simulink library "dspvect2"  (Simulink 3.00)
libraries: dspvect2 x2
settings Model: Creator=don  LastModifiedBy=tjones

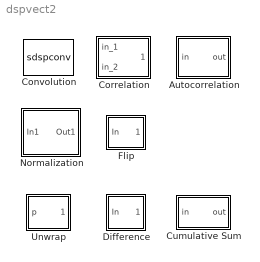
== system dspvect2 ==
  Autocorrelation : Subsystem  mask(Autocorrelation){maxlag=-1, bias=None}
      mask prompts: maxlag "Maximum positive lag (-1 for all positive lags)"; bias "Scaling:"
      mask help: Computes the autocorrelation function for non-negative lags in the range [0, length(u)-1].
      mask Help: web(dspbhelp);
      mask StyleString: edit,popup(None|Biased|Unbiased|Unity at zero-lag)
      mask Display: disp('ACF')
  Convolution : S-Function  FunctionName=sdspconv  PortCounts=[]  SFunctionModules=''
      mask Type: Convolution
      mask Description: Convolve two vectors.
      mask Help: web(dspbhelp);
      mask Display: disp('Conv')
  Correlation : Subsystem
      mask Type: Correlation
      mask Description: Correlation between two vectors.
      mask Help: web(dspbhelp);
      mask Display: disp('Corr')
  Cumulative Sum : Subsystem
      mask Type: Cumulative Sum
      mask Description: Cumulative sum of input elements.
      mask Help: web(dspbhelp);
      mask Display: disp('cumsum')
  Difference : Subsystem
      mask Type: Difference
      mask Description: Difference between adjacent vector input elements.
      mask Help: web(dspbhelp);
      mask Display: disp('diff')
  Flip : Subsystem
      mask Type: Flip
      mask Description: Reverse order of vector elements.
      mask Help: web(dspbhelp);
      mask Display: plot(0,0,100,100,[47 40 40 47],[20 20 90 90],[53 60 60 53],[90 90 20 20],[75 76 81 80 73],[34 24 40 60 90],[83 76],[29 24],[19 30 19 19 26],[86 84 72 50 20],[29 30],[71 84])
  Normalization : Subsystem  mask(Normalization){NormType=Squared 2-norm, Bias=1e-10}
      mask prompts: NormType "Norm:"; Bias "Normalization bias:"
      mask help: Normalize each input element by the vector 2-norm, sqrt(u'u)+b, or by the squared 2-norm, u'u+b, where b is a bias used to protect against divide-by-zero.
      mask init:
      | x = [0 NaN 100 NaN 20 80 NaN 30 30 NaN 36 36 NaN 58 58 NaN 64 64];
      | y = [0 NaN 100 NaN 60 60 NaN 9 43 NaN 9 43 NaN 9 43 NaN 9 43];
      | if NormType==1, sqr_txt = ' '; else sqr_txt = '2'; end
      mask Help: web(dspbhelp);
      mask StyleString: popup(2-norm|Squared 2-norm),edit
      mask Display:
      | plot(x,y)
      | text(44,80,'u'); text(44,25,'u'); text(72,39,sqr_txt)
  Unwrap : Subsystem  mask(Unwrap){tol=pi}
      mask prompts: tol "Tolerance (radians):"
      mask help: Remove phase discontinuities greater than tolerance threshold.
      mask Help: web(dspbhelp);
      mask Display: plot(0,0,100,100,[16 16],[92 8],[8 92],[16 16],[16 48 48 80],[64 44 76 56],[64 64 58 64 70],[60 40 46 40 46],[69 82],[30 22],[],[],[52 65],[41 33])

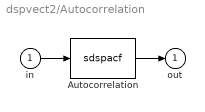
== system dspvect2/Autocorrelation ==
  in : Inport  Port=1  PortWidth=-1  SampleTime=-1  DataType=auto
      settings: SignalType=auto
  Autocorrelation : S-Function  FunctionName=sdspacf  Parameters=maxlag,bias  PortCounts=[]  SFunctionModules=''
  out : Outport  Port=1  InitialOutput=0
  wires:
  Autocorrelation/1 -> out/1
  in/1 -> Autocorrelation/1

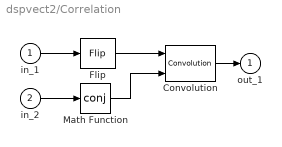
== system dspvect2/Correlation ==
  in_1 : Inport  Port=1  PortWidth=-1  SampleTime=-1  DataType=auto
      settings: SignalType=auto
  in_2 : Inport  Port=2  PortWidth=-1  SampleTime=-1  DataType=auto
      settings: SignalType=auto
  Convolution : dspvect2/Convolution
  Flip : dspvect2/Flip
  Math Function : Math  Operator=conj  OutputSignalType=auto
  out_1 : Outport  Port=1  InitialOutput=0
  wires:
  Convolution/1 -> out_1/1
  in_1/1 -> Flip/1
  Flip/1 -> Convolution/1
  in_2/1 -> Math Function/1
  Math Function/1 -> Convolution/2

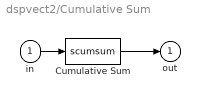
== system dspvect2/Cumulative Sum ==
  in : Inport  Port=1  PortWidth=-1  SampleTime=-1  DataType=auto
      settings: SignalType=auto
  Cumulative Sum : S-Function  FunctionName=scumsum  PortCounts=[]  SFunctionModules=''
  out : Outport  Port=1  InitialOutput=0
  wires:
  in/1 -> Cumulative Sum/1
  Cumulative Sum/1 -> out/1

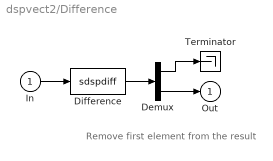
== system dspvect2/Difference ==
  note: Remove first element
      | from the result
  In : Inport  Port=1  PortWidth=-1  SampleTime=-1  DataType=auto
      settings: SignalType=auto
  Demux : Demux  Outputs=[1 -1]
  Difference : S-Function  FunctionName=sdspdiff  PortCounts=[]  SFunctionModules=''
  Terminator : Terminator
  Out : Outport  Port=1  InitialOutput=0
  wires:
  In/1 -> Difference/1
  Difference/1 -> Demux/1
  Demux/1 -> Terminator/1
  Demux/2 -> Out/1

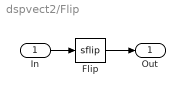
== system dspvect2/Flip ==
  In : Inport  Port=1  PortWidth=-1  SampleTime=-1  DataType=auto
      settings: SignalType=auto
  Flip : S-Function  FunctionName=sflip  PortCounts=[]  SFunctionModules=''
  Out : Outport  Port=1  InitialOutput=0
  wires:
  Flip/1 -> Out/1
  In/1 -> Flip/1

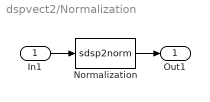
== system dspvect2/Normalization ==
  In1 : Inport  Port=1  PortWidth=-1  SampleTime=-1  DataType=auto
      settings: SignalType=auto
  Normalization : S-Function  FunctionName=sdsp2norm  Parameters=Bias,NormType  PortCounts=[]  SFunctionModules=''
  Out1 : Outport  Port=1  InitialOutput=0
  wires:
  In1/1 -> Normalization/1
  Normalization/1 -> Out1/1

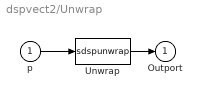
== system dspvect2/Unwrap ==
  p : Inport  Port=1  PortWidth=-1  SampleTime=-1  DataType=auto
      settings: SignalType=auto
  Unwrap : S-Function  FunctionName=sdspunwrap  Parameters=tol  PortCounts=[]  SFunctionModules=''
  Outport : Outport  Port=1  InitialOutput=0
  wires:
  Unwrap/1 -> Outport/1
  p/1 -> Unwrap/1
